simulink model "ES208A_CurrMeasArbn"  (R2013b)
settings: Solver=ode3  StartTime=0.0  StopTime=2  FixedStep=.000125  RelTol=1e-3
values from neighbouring files (symbols this model uses):
  CORRLNSTSCOMPCON1_ULS_U08 = DataDict.Constant    [ES208A_CurrMeasArbn_DataDict.m]
  CORRLNSTSCOMPCON2_ULS_U08 = DataDict.Constant    [ES208A_CurrMeasArbn_DataDict.m]
  CurrMeasArbnMaxStallCntr = DataDict.Calibration    [ES208A_CurrMeasArbn_DataDict.m]
  MOTCURRDAXQAXLIM_AMPR_F32 = DataDict.Constant    [ES208A_CurrMeasArbn_DataDict.m]
  ONEDIV3_ULS_F32 = DataDict.Constant    [ES208A_CurrMeasArbn_DataDict.m]
  ONEDIVSQRT3_ULS_F32 = DataDict.Constant    [ES208A_CurrMeasArbn_DataDict.m]
libraries: simulink x6
settings Model: Creator=hzy4g9  LastModifiedBy=hzy4g9
settings DebuggingCC: ParameterOverflowMsg=none

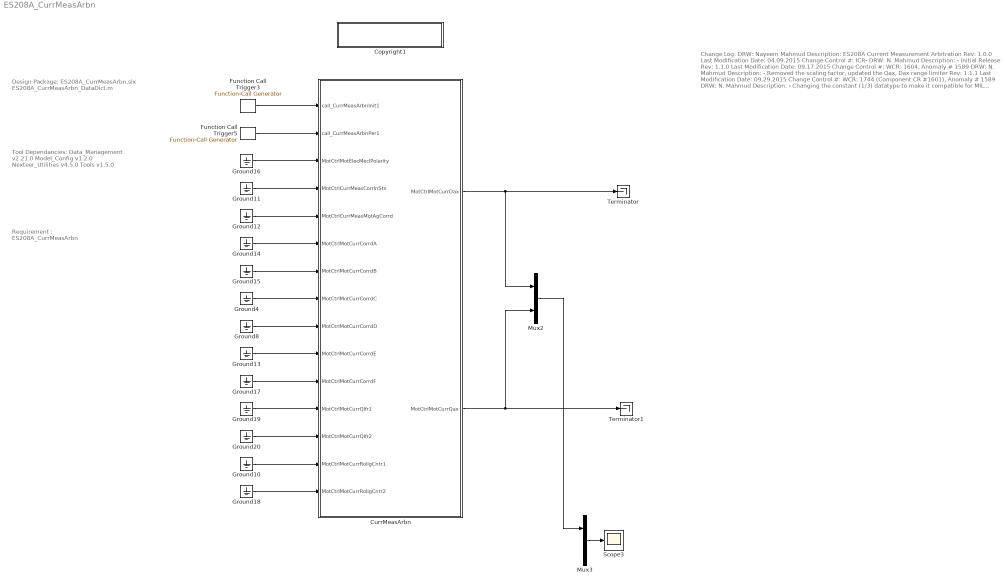
== system ES208A_CurrMeasArbn ==
  note: Design Package:
      |
      | ES208A_CurrMeasArbn.slx
      | ES208A_CurrMeasArbn_DataDict.m
  note: Tool Dependancies:
      |
      | Data_Management v2.21.0
      | Model_Config v1.2.0
      | Nexteer_Utilities v4.5.0
      | Tools v1.5.0
  note: Requirement :
      |
      | ES208A_CurrMeasArbn
  note: Change Log:
      |
      | DRW: Nayeem Mahmud
      | Description:
      | ES208A Current Measurement Arbitration
      |
      | Rev: 1.0.0
      | Last Modification Date: 04.09.2015
      | Change Control #: ICR-
      | DRW: N. Mahmud
      | Description:
      | - Initial Release
      |
      | Rev: 1.1.0
      | Last Modification Date: 09.17.2015
      | Change Control #: WCR: 1604, Anomaly # 1589
      | DRW: N. Mahmud
      | Description:
      | - Removed the scaling factor, updated the Qax, Dax range limiter
      |
      | Rev: 1.1.1
      | Last Modification Date: 09.29.2015
      | Change Control #: WCR: 1744 (Component CR #1601), Anomaly # 1589
      | DRW: N. Mahmud
      | Description:
      | - Changing the constant (1/3) datatype to make it compatible for MIL Testing.
      |
      |
      | Rev: 1.1.1
      | Last Modification Date: 09.29.2015
      | Change Control #: WCR: 1744 (Component CR #1601), Anomaly # 1589
      | DRW: N. Mahmud
      | Description:
      | - Changing the constant (1/3) datatype to make it compatible for MIL Testing.
      |
      |
      | Rev: 1.2.0
      | Last Modification Date: 10.16.2015
      | Change Control #: WCR: 2039 (Component CR #2011), Anomaly # 1965
      | DRW: N. Mahmud
      | Description:
      | - Requirement linkage between FR and the model has been corrected according the the MIL test review.
      | - Details can be found in Muragesh's email on 10.06.2015
      |
      |
      | Rev: 1.3.0
      | Last Modification Date: 03.15.2016
      | Change Control #: Anomaly # EA4#2989     Comp   EA4#4532	     WCR # EA4#4751
      | DRW: N. Mahmud
      | Description:
      | - Fixed the datatype mismatch on CurrMeasCorrlnSts connection
  Copyright1 : Subsystem  Description=|  mask(Copyright Information){none=on}
      | Copyright info block.                                               
      |                                                                     
      | Place copyright information at the top of every subsystem in design.
      mask prompts: none "No parameters"
      mask help: Place copyright information at the top of every subsystem in design.
      mask Display:
      | NxtrConf = 'Nexteer Confidential';
      | 
      | sys = bdroot; %handle for the current model ("system")
      | first = get_param(sys,'Created');
      | if(isempty(first))
      |     first = datestr(now,'yyyy');
      | else
      |     first = first(end-3:end);  %year is last four digits
      | end
      | 
      | last = get_param(sys,'LastModifiedDate');
      | if isempty(last)
      |     last = datestr(now,'yyyy');
      | else
      |     last = last(end-3:end);
      | end
      | 
      | if strcmp(first,last)
      |     fprintf('%s\nCopyright  %s Nexteer',NxtrConf,first);
      | else
      |     fprintf('%s\n%s%s-%s Nexteer',NxtrConf,char(169),first,last);
      | end
  CurrMeasArbn : Subsystem  RequirementInfo={} %GIDa_a1717183_1af4_4d60_b453_ff5ac2b3c2e1
  Function Call Trigger3 : simulink/Ports & Subsystems/Function-Call Generator  RequirementInfo={} %GIDa_b2c5acfa_4dcb_4ad4_8951_e2fcc0578f85  sample_time=0  numberOfIterations=1
  Function Call Trigger5 : simulink/Ports & Subsystems/Function-Call Generator  RequirementInfo={} %GIDa_0decdd2a_d3f7_4f78_a697_e4983ae5479f  sample_time=0.000125  numberOfIterations=1
  Ground{4,8,10..20} (13 alike) : Ground
  Mux2 : Mux  Inputs=2
  Mux3 : Mux  Inputs=2
  Scope3 : Scope
      settings: TimeRange=2  YMin=-70  YMax=70  SaveName=ScopeData6
  Terminator : Terminator
  Terminator1 : Terminator
  wires:
  Mux2/1 -> Mux3/1
  CurrMeasArbn/2(MotCtrlMotCurrQax) -> Mux2/2, Terminator1/1
  CurrMeasArbn/1(MotCtrlMotCurrDax) -> Terminator/1, Mux2/1
  Mux3/1 -> Scope3/1
  Function Call Trigger3/1 -> CurrMeasArbn/1(call_CurrMeasArbnInit1)
  Function Call Trigger5/1 -> CurrMeasArbn/2(call_CurrMeasArbnPer1)
  Ground18/1 -> CurrMeasArbn/15(MotCtrlMotCurrRollgCntr2)
  Ground20/1 -> CurrMeasArbn/13(MotCtrlMotCurrQlfr2)
  Ground10/1 -> CurrMeasArbn/14(MotCtrlMotCurrRollgCntr1)
  Ground14/1 -> CurrMeasArbn/6(MotCtrlMotCurrCorrdA)
  Ground19/1 -> CurrMeasArbn/12(MotCtrlMotCurrQlfr1)
  Ground11/1 -> CurrMeasArbn/4(MotCtrlCurrMeasCorrlnSts)
  Ground16/1 -> CurrMeasArbn/3(MotCtrlMotElecMeclPolarity)
  Ground12/1 -> CurrMeasArbn/5(MotCtrlCurrMeasMotAgCorrd)
  Ground4/1 -> CurrMeasArbn/8(MotCtrlMotCurrCorrdC)
  Ground17/1 -> CurrMeasArbn/11(MotCtrlMotCurrCorrdF)
  Ground8/1 -> CurrMeasArbn/9(MotCtrlMotCurrCorrdD)
  Ground13/1 -> CurrMeasArbn/10(MotCtrlMotCurrCorrdE)
  Ground15/1 -> CurrMeasArbn/7(MotCtrlMotCurrCorrdB)

== system ES208A_CurrMeasArbn/Copyright1 ==

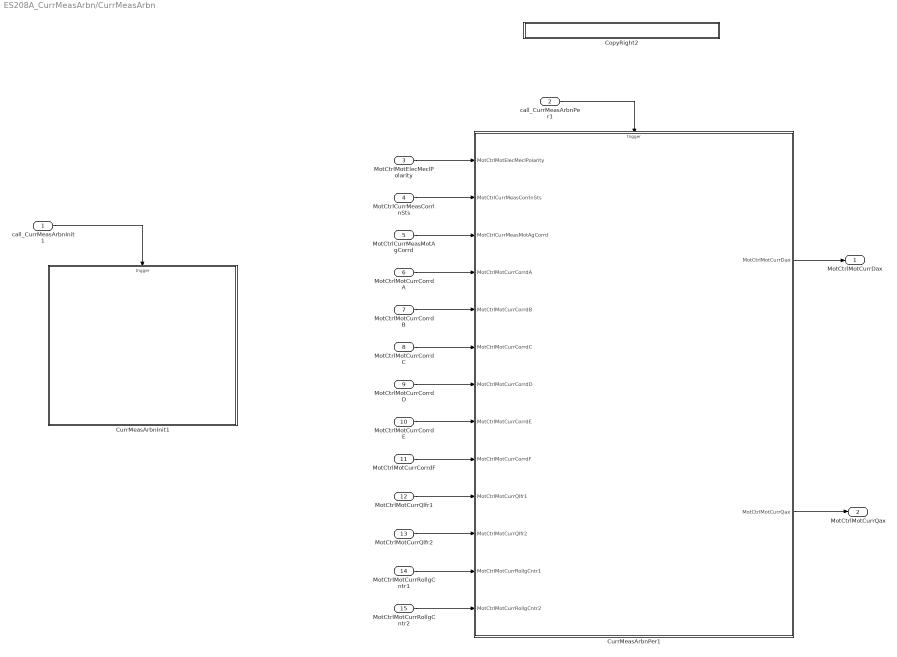
== system ES208A_CurrMeasArbn/CurrMeasArbn ==
  call_CurrMeasArbnInit1 : Inport
  call_CurrMeasArbnPer1 : Inport  Port=2
  MotCtrlMotElecMeclPolarity : Inport  RequirementInfo={'linktype_rmi_doors' '0000c363 (/ESG Group/FDD Module Requirements/EA4 Specific/ES208A CurrMeasArbn)' '#ES208A_200' 'true' 'REQ: ES208A_200' '' } %GIDa_2b3b6ccf_6739_4b84_95f8_6a6981087fde  Port=3
  MotCtrlCurrMeasCorrlnSts : Inport  RequirementInfo={'linktype_rmi_doors' '0000c363 (/ESG Group/FDD Module Requirements/EA4 Specific/ES208A CurrMeasArbn)' '#ES208A_205' 'true' 'REQ: ES208A_205' '' } %GIDa_b47cd3a1_346e_4c9b_a755_1899bf4f1f90  Port=4  OutDataTypeStr=uint16
  MotCtrlCurrMeasMotAgCorrd : Inport  RequirementInfo={'linktype_rmi_doors' '0000c363 (/ESG Group/FDD Module Requirements/EA4 Specific/ES208A CurrMeasArbn)' '#ES208A_202' 'true' 'REQ: ES208A_202' '' } %GIDa_3e28adf7_2d4b_4fb8_a0eb_8bdd2948163c  Port=5
  MotCtrlMotCurrCorrdA : Inport  RequirementInfo={'linktype_rmi_doors' '0000c363 (/ESG Group/FDD Module Requirements/EA4 Specific/ES208A CurrMeasArbn)' '#ES208A_104' 'true' 'REQ: ES208A_104' '' } %GIDa_fa60b5af_feb4_4057_8a17_b1f1cd5e1840  Port=6
  MotCtrlMotCurrCorrdB : Inport  RequirementInfo={'linktype_rmi_doors' '0000c363 (/ESG Group/FDD Module Requirements/EA4 Specific/ES208A CurrMeasArbn)' '#ES208A_103' 'true' 'REQ: ES208A_103' '' } %GIDa_236fb9c2_37b3_44dd_950c_8b8dc24ebe1f  Port=7
  MotCtrlMotCurrCorrdC : Inport  RequirementInfo={'linktype_rmi_doors' '0000c363 (/ESG Group/FDD Module Requirements/EA4 Specific/ES208A CurrMeasArbn)' '#ES208A_102' 'true' 'REQ: ES208A_102' '' } %GIDa_cb87798d_9ed2_4f24_a94d_155ef6f739fe  Port=8
  MotCtrlMotCurrCorrdD : Inport  RequirementInfo={'linktype_rmi_doors' '0000c363 (/ESG Group/FDD Module Requirements/EA4 Specific/ES208A CurrMeasArbn)' '#ES208A_101' 'true' 'REQ: ES208A_101' '' } %GIDa_061ae548_4f5f_4f77_9e99_bc9a7a97246f  Port=9
  MotCtrlMotCurrCorrdE : Inport  RequirementInfo={'linktype_rmi_doors' '0000c363 (/ESG Group/FDD Module Requirements/EA4 Specific/ES208A CurrMeasArbn)' '#ES208A_100' 'true' 'REQ: ES208A_100' '' } %GIDa_a1510a61_0232_4d8b_b15e_5251ba81e48f  Port=10
  MotCtrlMotCurrCorrdF : Inport  RequirementInfo={'linktype_rmi_doors' '0000c363 (/ESG Group/FDD Module Requirements/EA4 Specific/ES208A CurrMeasArbn)' '#ES208A_99' 'true' 'REQ: ES208A_99' '' } %GIDa_55e2ee94_269a_4388_9a08_e4c1affacd3d  Port=11
  MotCtrlMotCurrQlfr1 : Inport  RequirementInfo={'linktype_rmi_doors' '0000c363 (/ESG Group/FDD Module Requirements/EA4 Specific/ES208A CurrMeasArbn)' '#ES208A_215' 'true' 'REQ: ES208A_215' '' } %GIDa_d01b7b7a_10d2_4143_9f7b_655c2bbf76c3  Port=12
  MotCtrlMotCurrQlfr2 : Inport  RequirementInfo={'linktype_rmi_doors' '0000c363 (/ESG Group/FDD Module Requirements/EA4 Specific/ES208A CurrMeasArbn)' '#ES208A_214' 'true' 'REQ: ES208A_214' '' } %GIDa_a588847a_814e_4cd9_8192_8cc5b2289da5  Port=13
  MotCtrlMotCurrRollgCntr1 : Inport  RequirementInfo={'linktype_rmi_doors' '0000c363 (/ESG Group/FDD Module Requirements/EA4 Specific/ES208A CurrMeasArbn)' '#ES208A_213' 'true' 'REQ: ES208A_213' '' } %GIDa_81545b02_05c2_4ea8_b385_fe805407db0a  Port=14
  MotCtrlMotCurrRollgCntr2 : Inport  RequirementInfo={'linktype_rmi_doors' '0000c363 (/ESG Group/FDD Module Requirements/EA4 Specific/ES208A CurrMeasArbn)' '#ES208A_212' 'true' 'REQ: ES208A_212' '' } %GIDa_f58fb777_4bd7_43f0_8970_a93616277b47  Port=15
  CopyRight2 : Subsystem  Description=|  mask(Copyright Information){none=on}
      | Copyright info block.                                               
      |                                                                     
      | Place copyright information at the top of every subsystem in design.
      mask prompts: none "No parameters"
      mask help: Place copyright information at the top of every subsystem in design.
      mask Display:
      | NxtrConf = 'Nexteer Confidential';
      | 
      | sys = bdroot; %handle for the current model ("system")
      | first = get_param(sys,'Created');
      | first = first(end-3:end);  %year is last four digits
      | 
      | last = get_param(sys,'LastModifiedDate');
      | if isempty(last)
      |     last = datestr(now,'yyyy');
      | else
      |     last = last(end-3:end);
      | end
      | 
      | if strcmp(first,last)
      |     fprintf('%s -- Copyright %s Nexteer',NxtrConf,first)
      | else
      |     fprintf('%s -- %s%s- %s Nexteer',NxtrConf,char(169),first,last)
      | end
  CurrMeasArbnInit1 : Subsystem  RequirementInfo={'linktype_rmi_doors' '0000c363 (/ESG Group/FDD Module Requirements/EA4 Specific/ES208A CurrMeasArbn)' '#ES208A_216' 'true' 'REQ: ES208A_216' '' } %GIDa_4d08f95b_63fa_42b7_bb43_10901df62bca
  CurrMeasArbnPer1 : Subsystem  RequirementInfo={'linktype_rmi_doors' '0000c363 (/ESG Group/FDD Module Requirements/EA4 Specific/ES208A CurrMeasArbn)' '#ES208A_216' 'true' 'REQ: ES208A_216' '' } %GIDa_5d0a6b13_94ef_43df_a64b_8db993e8cc82
  MotCtrlMotCurrDax : Outport  RequirementInfo={'linktype_rmi_doors' '0000c363 (/ESG Group/FDD Module Requirements/EA4 Specific/ES208A CurrMeasArbn)' '#ES208A_204' 'true' 'REQ: ES208A_204' '' } %GIDa_641f96e7_6a3f_402c_952a_c727130605fe
  MotCtrlMotCurrQax : Outport  RequirementInfo={'linktype_rmi_doors' '0000c363 (/ESG Group/FDD Module Requirements/EA4 Specific/ES208A CurrMeasArbn)' '#ES208A_206' 'true' 'REQ: ES208A_206' '' } %GIDa_55e00c49_dae8_43a4_8cfe_81b053089442  Port=2
  wires:
  CurrMeasArbnPer1/1(MotCtrlMotCurrDax) -> MotCtrlMotCurrDax/1
  CurrMeasArbnPer1/2(MotCtrlMotCurrQax) -> MotCtrlMotCurrQax/1
  call_CurrMeasArbnPer1/1 -> CurrMeasArbnPer1/Trigger
  MotCtrlMotElecMeclPolarity/1 -> CurrMeasArbnPer1/1(MotCtrlMotElecMeclPolarity)
  MotCtrlCurrMeasCorrlnSts/1 -> CurrMeasArbnPer1/2(MotCtrlCurrMeasCorrlnSts)
  MotCtrlCurrMeasMotAgCorrd/1 -> CurrMeasArbnPer1/3(MotCtrlCurrMeasMotAgCorrd)
  MotCtrlMotCurrCorrdA/1 -> CurrMeasArbnPer1/4(MotCtrlMotCurrCorrdA)
  MotCtrlMotCurrCorrdB/1 -> CurrMeasArbnPer1/5(MotCtrlMotCurrCorrdB)
  MotCtrlMotCurrCorrdC/1 -> CurrMeasArbnPer1/6(MotCtrlMotCurrCorrdC)
  MotCtrlMotCurrCorrdD/1 -> CurrMeasArbnPer1/7(MotCtrlMotCurrCorrdD)
  MotCtrlMotCurrCorrdE/1 -> CurrMeasArbnPer1/8(MotCtrlMotCurrCorrdE)
  MotCtrlMotCurrCorrdF/1 -> CurrMeasArbnPer1/9(MotCtrlMotCurrCorrdF)
  MotCtrlMotCurrQlfr1/1 -> CurrMeasArbnPer1/10(MotCtrlMotCurrQlfr1)
  MotCtrlMotCurrQlfr2/1 -> CurrMeasArbnPer1/11(MotCtrlMotCurrQlfr2)
  MotCtrlMotCurrRollgCntr1/1 -> CurrMeasArbnPer1/12(MotCtrlMotCurrRollgCntr1)
  MotCtrlMotCurrRollgCntr2/1 -> CurrMeasArbnPer1/13(MotCtrlMotCurrRollgCntr2)
  call_CurrMeasArbnInit1/1 -> CurrMeasArbnInit1/Trigger

== system ES208A_CurrMeasArbn/CurrMeasArbn/CopyRight2 ==

== system ES208A_CurrMeasArbn/CurrMeasArbn/CurrMeasArbnInit1 ==
  note: Init function is added to have a RTE function associated with the periodic
      | which runs at motor control ISR rate so that Calibrations and PIMs can be
      | initialized/configured through RTE
  Trigger : TriggerPort  TriggerType=function-call  PortDimensions=1

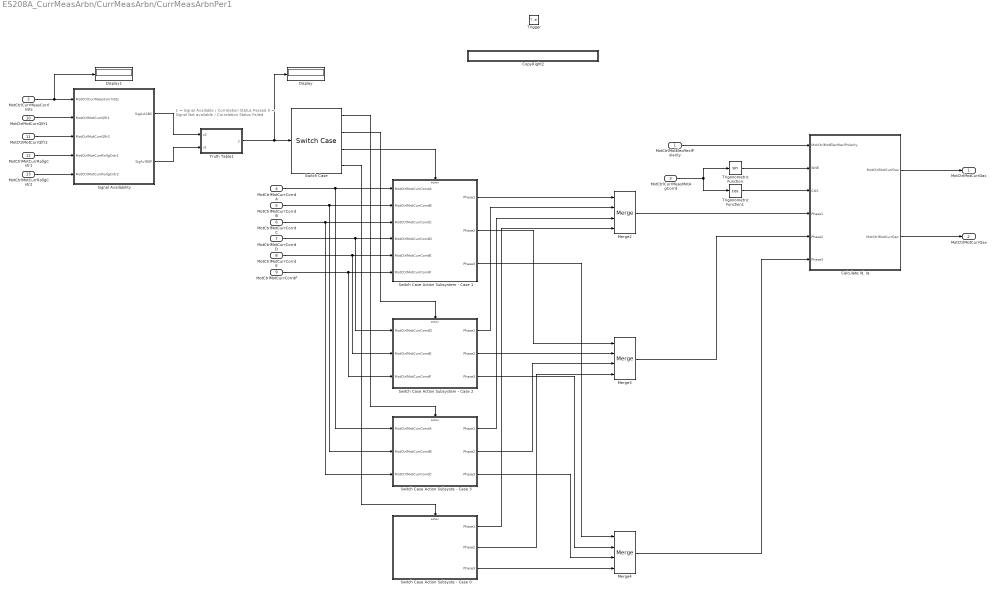
== system ES208A_CurrMeasArbn/CurrMeasArbn/CurrMeasArbnPer1 ==
  note: 1 = Signal Available / Correlation Status Passed
      | 0 = Signal Not available / Correlation Status Failed
  MotCtrlMotElecMeclPolarity : Inport  RequirementInfo={} %GIDa_236c7770_dbe0_4d6b_854a_af419427730c
  MotCtrlCurrMeasCorrlnSts : Inport  RequirementInfo={} %GIDa_5f0ff581_beb2_45c0_96fc_3ae60b8cafd0  Port=2
  MotCtrlCurrMeasMotAgCorrd : Inport  Port=3  OutDataTypeStr=single
  MotCtrlMotCurrCorrdA : Inport  RequirementInfo={} %GIDa_f9a6d725_8597_45da_8d5a_d49e87f1c418  Port=4
  MotCtrlMotCurrCorrdB : Inport  RequirementInfo={} %GIDa_4ecfd322_1f8c_4f95_b72b_4a4f2c3592db  Port=5
  MotCtrlMotCurrCorrdC : Inport  RequirementInfo={} %GIDa_50682985_192f_42e9_ab67_18d9d790db6a  Port=6
  MotCtrlMotCurrCorrdD : Inport  RequirementInfo={} %GIDa_08227d3c_7fbb_46ed_9d72_22bcb1c5ff3a  Port=7
  MotCtrlMotCurrCorrdE : Inport  RequirementInfo={} %GIDa_5724e0f4_ed90_4089_ab16_14491ea93933  Port=8
  MotCtrlMotCurrCorrdF : Inport  RequirementInfo={} %GIDa_7a043740_7caa_40bd_b933_0baae6bc5fb0  Port=9
  MotCtrlMotCurrQlfr1 : Inport  RequirementInfo={} %GIDa_d0b4e530_bfd9_4c60_aa9a_209d86ff3bd1  Port=10
  MotCtrlMotCurrQlfr2 : Inport  RequirementInfo={} %GIDa_775a9752_c098_48a0_adc4_e5952c0b608a  Port=11
  MotCtrlMotCurrRollgCntr1 : Inport  RequirementInfo={} %GIDa_059ee444_07c8_42c9_bb13_b03c4afc962a  Port=12
  MotCtrlMotCurrRollgCntr2 : Inport  RequirementInfo={} %GIDa_23ffabf9_7016_4a97_b10a_a8e5452610f9  Port=13  OutDataTypeStr=uint8
  Trigger : TriggerPort  TriggerType=function-call  PortDimensions=1
  "Calculate Id, Iq" : Subsystem  RequirementInfo={'linktype_rmi_doors' '0000c363 (/ESG Group/FDD Module Requirements/EA4 Specific/ES208A CurrMeasArbn)' '#ES208A_15' 'true' 'REQ: ES208A_15' '' ; 'linktype_rmi_doors' '0000c363 (/ESG Group/FDD Module Requirements/EA4 Specific/ES208A CurrMeasArbn)' '#ES208A_221' 'true' 'REQ: ES208A_221' '' } %GIDa_d3675425_55ad_4442_a97f_0532e8744e77
  CopyRight2 : Subsystem  Description=|  mask(Copyright Information){none=on}
      | Copyright info block.                                               
      |                                                                     
      | Place copyright information at the top of every subsystem in design.
      mask prompts: none "No parameters"
      mask help: Place copyright information at the top of every subsystem in design.
      mask Display:
      | NxtrConf = 'Nexteer Confidential';
      | 
      | sys = bdroot; %handle for the current model ("system")
      | first = get_param(sys,'Created');
      | first = first(end-3:end);  %year is last four digits
      | 
      | last = get_param(sys,'LastModifiedDate');
      | if isempty(last)
      |     last = datestr(now,'yyyy');
      | else
      |     last = last(end-3:end);
      | end
      | 
      | if strcmp(first,last)
      |     fprintf('%s -- Copyright %s Nexteer',NxtrConf,first)
      | else
      |     fprintf('%s -- %s%s- %s Nexteer',NxtrConf,char(169),first,last)
      | end
  Display : Display
  Display1 : Display
  Merge2 : Merge  Inputs=4
  Merge3 : Merge  Inputs=4
  Merge4 : Merge  Inputs=4
  Signal Availability : Subsystem  RequirementInfo={} %GIDa_5e4be01c_85da_4430_af9b_2a4846b816f0
  Switch Case : SwitchCase  CaseConditions={3,2,1}
  Switch Case Action Subsyste - Case 0 : Subsystem  RequirementInfo={'linktype_rmi_doors' '0000c363 (/ESG Group/FDD Module Requirements/EA4 Specific/ES208A CurrMeasArbn)' '#ES208A_220' 'true' 'REQ: ES208A_220' '' } %GIDa_4f294f1a_407e_4985_88ae_1f48918d334e  TreatAsAtomicUnit=on
  Switch Case Action Subsyste - Case 3 : Subsystem  RequirementInfo={'linktype_rmi_doors' '0000c363 (/ESG Group/FDD Module Requirements/EA4 Specific/ES208A CurrMeasArbn)' '#ES208A_217' 'true' 'REQ: ES208A_217' '' } %GIDa_710d68b6_e234_43e9_bbdb_b14f4ce7fdcf  TreatAsAtomicUnit=on
  Switch Case Action Subsystem - Case 1 : Subsystem  RequirementInfo={'linktype_rmi_doors' '0000c363 (/ESG Group/FDD Module Requirements/EA4 Specific/ES208A CurrMeasArbn)' '#ES208A_211' 'true' 'REQ: ES208A_211' '' } %GIDa_4f02c82c_3123_42cc_bef6_8026bf4aaa33  TreatAsAtomicUnit=on
  Switch Case Action Subsystem - Case 2 : Subsystem  RequirementInfo={'linktype_rmi_doors' '0000c363 (/ESG Group/FDD Module Requirements/EA4 Specific/ES208A CurrMeasArbn)' '#ES208A_218' 'true' 'REQ: ES208A_218' '' } %GIDa_61ae6b1b_e240_4075_bddf_edb8f2fb6854  TreatAsAtomicUnit=on
  Trigonometric Function : Trigonometry
  Trigonometric Function1 : Trigonometry  Operator=cos
  Truth Table1 : Truth Table  TreatAsAtomicUnit=on
  MotCtrlMotCurrDax : Outport  RequirementInfo={} %GIDa_fc90444e_e698_458a_bc45_6a75ea4d8c72
  MotCtrlMotCurrQax : Outport  RequirementInfo={} %GIDa_65000aaa_3595_4279_a6c5_6d4c8a6042b5  Port=2
  wires:
  Truth Table1/1(y) -> Display/1, Switch Case/1
  MotCtrlCurrMeasMotAgCorrd/1 -> Trigonometric Function1/1, Trigonometric Function/1
  Switch Case/3 -> Switch Case Action Subsystem - Case 1/Action
  Switch Case/2 -> Switch Case Action Subsystem - Case 2/Action
  MotCtrlCurrMeasCorrlnSts/1 -> Signal Availability/1(MotCtrlCurrMeasCorrlnSts), Display1/1
  MotCtrlMotCurrQlfr2/1 -> Signal Availability/3(MotCtrlMotCurrQlfr2)
  MotCtrlMotCurrRollgCntr2/1 -> Signal Availability/5(MotCtrlMotCurrRollgCntr2)
  MotCtrlMotCurrQlfr1/1 -> Signal Availability/2(MotCtrlMotCurrQlfr1)
  MotCtrlMotCurrRollgCntr1/1 -> Signal Availability/4(MotCtrlMotCurrRollgCntr1)
  Signal Availability/1(SigAvlABC) -> Truth Table1/1(u2)
  Signal Availability/2("SigAvlDEF ") -> Truth Table1/2(u1)
  Switch Case/4 -> Switch Case Action Subsyste - Case 0/Action
  Switch Case/1 -> Switch Case Action Subsyste - Case 3/Action
  MotCtrlMotCurrCorrdC/1 -> Switch Case Action Subsyste - Case 3/3(MotCtrlMotCurrCorrdC), Switch Case Action Subsystem - Case 1/3(MotCtrlMotCurrCorrdC)
  MotCtrlMotCurrCorrdB/1 -> Switch Case Action Subsyste - Case 3/2(MotCtrlMotCurrCorrdB), Switch Case Action Subsystem - Case 1/2(MotCtrlMotCurrCorrdB)
  MotCtrlMotCurrCorrdA/1 -> Switch Case Action Subsyste - Case 3/1(MotCtrlMotCurrCorrdA), Switch Case Action Subsystem - Case 1/1(MotCtrlMotCurrCorrdA)
  MotCtrlMotCurrCorrdF/1 -> Switch Case Action Subsystem - Case 2/3(MotCtrlMotCurrCorrdF), Switch Case Action Subsystem - Case 1/6(MotCtrlMotCurrCorrdF)
  MotCtrlMotCurrCorrdD/1 -> Switch Case Action Subsystem - Case 2/1(MotCtrlMotCurrCorrdD), Switch Case Action Subsystem - Case 1/4(MotCtrlMotCurrCorrdD)
  MotCtrlMotCurrCorrdE/1 -> Switch Case Action Subsystem - Case 2/2(MotCtrlMotCurrCorrdE), Switch Case Action Subsystem - Case 1/5(MotCtrlMotCurrCorrdE)
  Switch Case Action Subsystem - Case 1/1(Phase1) -> Merge2/1
  Switch Case Action Subsystem - Case 2/1(Phase1) -> Merge2/2
  Switch Case Action Subsyste - Case 3/1(Phase1) -> Merge2/3
  Switch Case Action Subsyste - Case 0/1(Phase1) -> Merge2/4
  Switch Case Action Subsystem - Case 1/2(Phase2) -> Merge3/1
  Switch Case Action Subsystem - Case 2/2(Phase2) -> Merge3/2
  Switch Case Action Subsyste - Case 3/2(Phase2) -> Merge3/3
  Switch Case Action Subsyste - Case 0/2(Phase2) -> Merge3/4
  Switch Case Action Subsystem - Case 1/3(Phase3) -> Merge4/1
  Switch Case Action Subsystem - Case 2/3(Phase3) -> Merge4/2
  Switch Case Action Subsyste - Case 3/3(Phase3) -> Merge4/3
  Switch Case Action Subsyste - Case 0/3(Phase3) -> Merge4/4
  "Calculate Id, Iq"/1(MotCtrlMotCurrDax) -> MotCtrlMotCurrDax/1
  "Calculate Id, Iq"/2(MotCtrlMotCurrQax) -> MotCtrlMotCurrQax/1
  Trigonometric Function/1 -> "Calculate Id, Iq"/2(SINE)
  Trigonometric Function1/1 -> "Calculate Id, Iq"/3(COS)
  MotCtrlMotElecMeclPolarity/1 -> "Calculate Id, Iq"/1(MotCtrlMotElecMeclPolarity)
  Merge2/1 -> "Calculate Id, Iq"/4(Phase1)
  Merge3/1 -> "Calculate Id, Iq"/5(Phase2)
  Merge4/1 -> "Calculate Id, Iq"/6(Phase3)

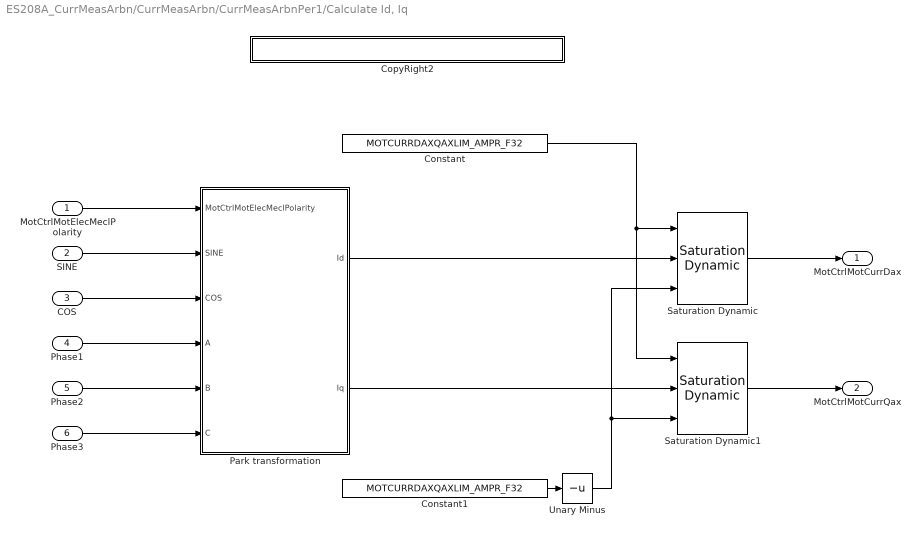
== system ES208A_CurrMeasArbn/CurrMeasArbn/CurrMeasArbnPer1/Calculate Id, Iq ==
  MotCtrlMotElecMeclPolarity : Inport  RequirementInfo={} %GIDa_f0c87258_af0d_44ef_b166_709dccf31a80
  SINE : Inport  Port=2
  COS : Inport  Port=3
  Phase1 : Inport  Port=4  OutDataTypeStr=single
  Phase2 : Inport  Port=5  OutDataTypeStr=single
  Phase3 : Inport  Port=6  OutDataTypeStr=single
  Constant : Constant  Value=MOTCURRDAXQAXLIM_AMPR_F32
  Constant1 : Constant  Value=MOTCURRDAXQAXLIM_AMPR_F32
  CopyRight2 : Subsystem  Description=|  mask(Copyright Information){none=on}
      | Copyright info block.                                               
      |                                                                     
      | Place copyright information at the top of every subsystem in design.
      mask prompts: none "No parameters"
      mask help: Place copyright information at the top of every subsystem in design.
      mask Display:
      | NxtrConf = 'Nexteer Confidential';
      | 
      | sys = bdroot; %handle for the current model ("system")
      | first = get_param(sys,'Created');
      | first = first(end-3:end);  %year is last four digits
      | 
      | last = get_param(sys,'LastModifiedDate');
      | if isempty(last)
      |     last = datestr(now,'yyyy');
      | else
      |     last = last(end-3:end);
      | end
      | 
      | if strcmp(first,last)
      |     fprintf('%s -- Copyright %s Nexteer',NxtrConf,first)
      | else
      |     fprintf('%s -- %s%s- %s Nexteer',NxtrConf,char(169),first,last)
      | end
  Park transformation : Subsystem  RequirementInfo={'linktype_rmi_doors' '0000c363 (/ESG Group/FDD Module Requirements/EA4 Specific/ES208A CurrMeasArbn)' '#ES208A_221' 'true' 'REQ: ES208A_221' '' } %GIDa_d3ede396_e304_4918_89ce_5b6c0de97769
  Saturation Dynamic : simulink/Discontinuities/Saturation Dynamic  RequirementInfo={'linktype_rmi_doors' '0000c363 (/ESG Group/FDD Module Requirements/EA4 Specific/ES208A CurrMeasArbn)' '#ES208A_222' 'true' 'REQ: ES208A_222' '' } %GIDa_6e2e1fe4_dfc6_46e0_b1ff_e247798a13b4  OutMin=[]  OutMax=[]  OutDataTypeStr=Inherit: Same as second input  OutDataType=fixdt(1, 16)  OutScaling=2^-10  DoSatur=off
  Saturation Dynamic1 : simulink/Discontinuities/Saturation Dynamic  RequirementInfo={'linktype_rmi_doors' '0000c363 (/ESG Group/FDD Module Requirements/EA4 Specific/ES208A CurrMeasArbn)' '#ES208A_222' 'true' 'REQ: ES208A_222' '' } %GIDa_ef7f06fc_ceb7_4b34_a03b_affe5dfaca83  OutMin=[]  OutMax=[]  OutDataTypeStr=Inherit: Same as second input  OutDataType=fixdt(1, 16)  OutScaling=2^-10  DoSatur=off
  Unary Minus : UnaryMinus
  MotCtrlMotCurrDax : Outport
  MotCtrlMotCurrQax : Outport  Port=2
  wires:
  Phase2/1 -> Park transformation/5(B)
  Phase3/1 -> Park transformation/6(C)
  Phase1/1 -> Park transformation/4(A)
  MotCtrlMotElecMeclPolarity/1 -> Park transformation/1(MotCtrlMotElecMeclPolarity)
  SINE/1 -> Park transformation/2(SINE)
  COS/1 -> Park transformation/3(COS)
  Park transformation/1(Id) -> Saturation Dynamic/2
  Park transformation/2(Iq) -> Saturation Dynamic1/2
  Saturation Dynamic/1 -> MotCtrlMotCurrDax/1
  Saturation Dynamic1/1 -> MotCtrlMotCurrQax/1
  Constant/1 -> Saturation Dynamic/1, Saturation Dynamic1/1
  Unary Minus/1 -> Saturation Dynamic/3, Saturation Dynamic1/3
  Constant1/1 -> Unary Minus/1

== system ES208A_CurrMeasArbn/CurrMeasArbn/CurrMeasArbnPer1/CopyRight2 ==

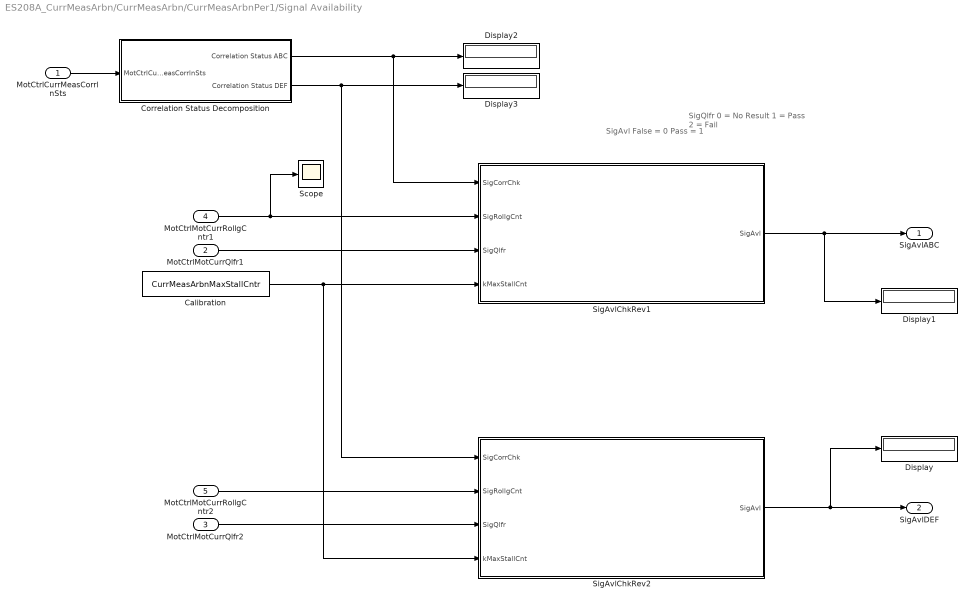
== system ES208A_CurrMeasArbn/CurrMeasArbn/CurrMeasArbnPer1/Signal Availability ==
  note: SigQlfr
      | 0 = No Result
      | 1 = Pass
      | 2 = Fail
  note: SigAvl
      | False = 0
      | Pass = 1
  MotCtrlCurrMeasCorrlnSts : Inport
  MotCtrlMotCurrQlfr1 : Inport  RequirementInfo={} %GIDa_edd0a4a8_ec9a_4294_bd7b_dc00380f4e82  Port=2
  MotCtrlMotCurrQlfr2 : Inport  RequirementInfo={} %GIDa_39258a34_15c4_42b2_b2a5_87a9df44d1d3  Port=3
  MotCtrlMotCurrRollgCntr1 : Inport  RequirementInfo={} %GIDa_9fc2b2d5_9d4a_4481_bff5_db7bbf1f5598  Port=4
  MotCtrlMotCurrRollgCntr2 : Inport  RequirementInfo={} %GIDa_1cde4ce6_8634_4cd8_b985_cde8bd6e892e  Port=5
  Calibration : Constant  Value=CurrMeasArbnMaxStallCntr
  "Correlation Status Decomposition " : Subsystem  RequirementInfo={'linktype_rmi_doors' '0000c363 (/ESG Group/FDD Module Requirements/EA4 Specific/ES208A CurrMeasArbn)' '#ES208A_135' 'true' 'REQ: ES208A_135' '' ; 'linktype_rmi_doors' '0000c363 (/ESG Group/FDD Module Requirements/EA4 Specific/ES208A CurrMeasArbn)' '#ES208A_219' 'true' 'REQ: ES208A_219' '' } %GIDa_c140fad4_ae0f_42b6_91b3_b7b2268b2aab
  Display{,1..3} (4 alike) : Display
  Scope : Scope
  SigAvlChkRev1 : Subsystem  RequirementInfo={'linktype_rmi_doors' '0000c363 (/ESG Group/FDD Module Requirements/EA4 Specific/ES208A CurrMeasArbn)' '#ES208A_135' 'true' 'REQ: ES208A_135' '' } %GIDa_b2a9f5a1_8dd0_41b9_a883_77a286bcb317  TreatAsAtomicUnit=on
  SigAvlChkRev2 : Subsystem  RequirementInfo={'linktype_rmi_doors' '0000c363 (/ESG Group/FDD Module Requirements/EA4 Specific/ES208A CurrMeasArbn)' '#ES208A_219' 'true' 'REQ: ES208A_219' '' } %GIDa_bf4ef0a2_bb1f_46f7_985b_0b0c9d147fc2  TreatAsAtomicUnit=on
  SigAvlABC : Outport
  "SigAvlDEF " : Outport  Port=2
  wires:
  MotCtrlCurrMeasCorrlnSts/1 -> "Correlation Status Decomposition "/1(MotCtrlCurrMeasCorrlnSts)
  "Correlation Status Decomposition "/1(Correlation Status ABC) -> SigAvlChkRev1/1(SigCorrChk), Display2/1
  MotCtrlMotCurrRollgCntr1/1 -> SigAvlChkRev1/2(SigRollgCnt), Scope/1
  MotCtrlMotCurrQlfr1/1 -> SigAvlChkRev1/3(SigQlfr)
  "Correlation Status Decomposition "/2(Correlation Status DEF) -> SigAvlChkRev2/1(SigCorrChk), Display3/1
  MotCtrlMotCurrRollgCntr2/1 -> SigAvlChkRev2/2(SigRollgCnt)
  MotCtrlMotCurrQlfr2/1 -> SigAvlChkRev2/3(SigQlfr)
  Calibration/1 -> SigAvlChkRev2/4(kMaxStallCnt), SigAvlChkRev1/4(kMaxStallCnt)
  SigAvlChkRev2/1(SigAvl) -> Display/1, "SigAvlDEF "/1
  SigAvlChkRev1/1(SigAvl) -> SigAvlABC/1, Display1/1

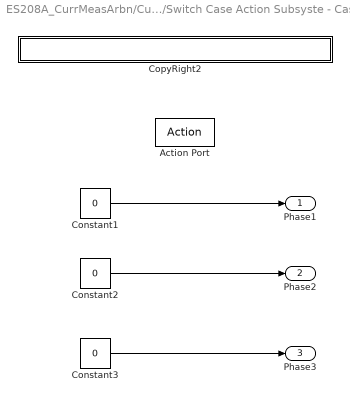
== system ES208A_CurrMeasArbn/CurrMeasArbn/CurrMeasArbnPer1/Switch Case Action Subsyste - Case 0 ==
  Action Port : ActionPort  ActionType=default
  Constant1 : Constant  Value=0  OutDataTypeStr=single
  Constant2 : Constant  Value=0  OutDataTypeStr=single
  Constant3 : Constant  Value=0  OutDataTypeStr=single
  CopyRight2 : Subsystem  Description=|  mask(Copyright Information){none=on}
      | Copyright info block.                                               
      |                                                                     
      | Place copyright information at the top of every subsystem in design.
      mask prompts: none "No parameters"
      mask help: Place copyright information at the top of every subsystem in design.
      mask Display:
      | NxtrConf = 'Nexteer Confidential';
      | 
      | sys = bdroot; %handle for the current model ("system")
      | first = get_param(sys,'Created');
      | first = first(end-3:end);  %year is last four digits
      | 
      | last = get_param(sys,'LastModifiedDate');
      | if isempty(last)
      |     last = datestr(now,'yyyy');
      | else
      |     last = last(end-3:end);
      | end
      | 
      | if strcmp(first,last)
      |     fprintf('%s -- Copyright %s Nexteer',NxtrConf,first)
      | else
      |     fprintf('%s -- %s%s- %s Nexteer',NxtrConf,char(169),first,last)
      | end
  Phase1 : Outport
  Phase2 : Outport  Port=2
  Phase3 : Outport  Port=3
  wires:
  Constant2/1 -> Phase2/1
  Constant1/1 -> Phase1/1
  Constant3/1 -> Phase3/1

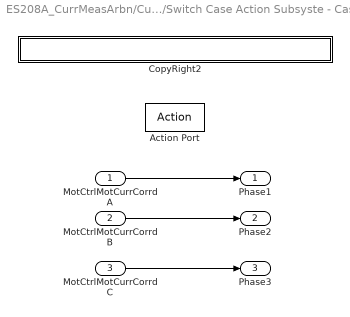
== system ES208A_CurrMeasArbn/CurrMeasArbn/CurrMeasArbnPer1/Switch Case Action Subsyste - Case 3 ==
  MotCtrlMotCurrCorrdA : Inport
  MotCtrlMotCurrCorrdB : Inport  Port=2
  MotCtrlMotCurrCorrdC : Inport  Port=3
  Action Port : ActionPort  ActionType=case
  CopyRight2 : Subsystem  Description=|  mask(Copyright Information){none=on}
      | Copyright info block.                                               
      |                                                                     
      | Place copyright information at the top of every subsystem in design.
      mask prompts: none "No parameters"
      mask help: Place copyright information at the top of every subsystem in design.
      mask Display:
      | NxtrConf = 'Nexteer Confidential';
      | 
      | sys = bdroot; %handle for the current model ("system")
      | first = get_param(sys,'Created');
      | first = first(end-3:end);  %year is last four digits
      | 
      | last = get_param(sys,'LastModifiedDate');
      | if isempty(last)
      |     last = datestr(now,'yyyy');
      | else
      |     last = last(end-3:end);
      | end
      | 
      | if strcmp(first,last)
      |     fprintf('%s -- Copyright %s Nexteer',NxtrConf,first)
      | else
      |     fprintf('%s -- %s%s- %s Nexteer',NxtrConf,char(169),first,last)
      | end
  Phase1 : Outport
  Phase2 : Outport  Port=2
  Phase3 : Outport  Port=3
  wires:
  MotCtrlMotCurrCorrdC/1 -> Phase3/1
  MotCtrlMotCurrCorrdB/1 -> Phase2/1
  MotCtrlMotCurrCorrdA/1 -> Phase1/1

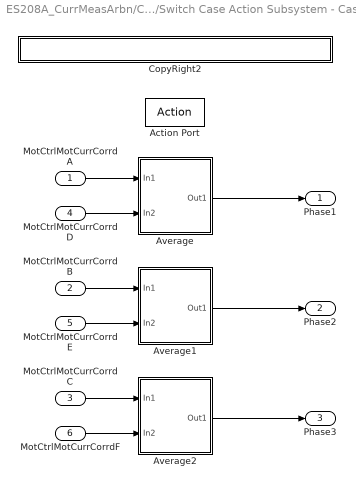
== system ES208A_CurrMeasArbn/CurrMeasArbn/CurrMeasArbnPer1/Switch Case Action Subsystem - Case 1 ==
  MotCtrlMotCurrCorrdA : Inport
  MotCtrlMotCurrCorrdB : Inport  Port=2
  MotCtrlMotCurrCorrdC : Inport  Port=3
  MotCtrlMotCurrCorrdD : Inport  Port=4
  MotCtrlMotCurrCorrdE : Inport  Port=5
  MotCtrlMotCurrCorrdF : Inport  Port=6
  Action Port : ActionPort  ActionType=case
  Average : Subsystem
  Average1 : Subsystem
  Average2 : Subsystem
  CopyRight2 : Subsystem  Description=|  mask(Copyright Information){none=on}
      | Copyright info block.                                               
      |                                                                     
      | Place copyright information at the top of every subsystem in design.
      mask prompts: none "No parameters"
      mask help: Place copyright information at the top of every subsystem in design.
      mask Display:
      | NxtrConf = 'Nexteer Confidential';
      | 
      | sys = bdroot; %handle for the current model ("system")
      | first = get_param(sys,'Created');
      | first = first(end-3:end);  %year is last four digits
      | 
      | last = get_param(sys,'LastModifiedDate');
      | if isempty(last)
      |     last = datestr(now,'yyyy');
      | else
      |     last = last(end-3:end);
      | end
      | 
      | if strcmp(first,last)
      |     fprintf('%s -- Copyright %s Nexteer',NxtrConf,first)
      | else
      |     fprintf('%s -- %s%s- %s Nexteer',NxtrConf,char(169),first,last)
      | end
  Phase1 : Outport
  Phase2 : Outport  Port=2
  Phase3 : Outport  Port=3
  wires:
  MotCtrlMotCurrCorrdA/1 -> Average/1(In1)
  MotCtrlMotCurrCorrdD/1 -> Average/2(In2)
  MotCtrlMotCurrCorrdE/1 -> Average1/2(In2)
  MotCtrlMotCurrCorrdB/1 -> Average1/1(In1)
  MotCtrlMotCurrCorrdF/1 -> Average2/2(In2)
  MotCtrlMotCurrCorrdC/1 -> Average2/1(In1)
  Average/1(Out1) -> Phase1/1
  Average2/1(Out1) -> Phase3/1
  Average1/1(Out1) -> Phase2/1

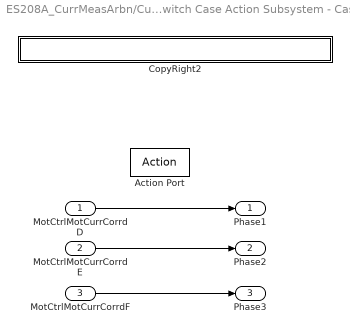
== system ES208A_CurrMeasArbn/CurrMeasArbn/CurrMeasArbnPer1/Switch Case Action Subsystem - Case 2 ==
  MotCtrlMotCurrCorrdD : Inport
  MotCtrlMotCurrCorrdE : Inport  Port=2
  MotCtrlMotCurrCorrdF : Inport  Port=3
  Action Port : ActionPort  ActionType=case
  CopyRight2 : Subsystem  Description=|  mask(Copyright Information){none=on}
      | Copyright info block.                                               
      |                                                                     
      | Place copyright information at the top of every subsystem in design.
      mask prompts: none "No parameters"
      mask help: Place copyright information at the top of every subsystem in design.
      mask Display:
      | NxtrConf = 'Nexteer Confidential';
      | 
      | sys = bdroot; %handle for the current model ("system")
      | first = get_param(sys,'Created');
      | first = first(end-3:end);  %year is last four digits
      | 
      | last = get_param(sys,'LastModifiedDate');
      | if isempty(last)
      |     last = datestr(now,'yyyy');
      | else
      |     last = last(end-3:end);
      | end
      | 
      | if strcmp(first,last)
      |     fprintf('%s -- Copyright %s Nexteer',NxtrConf,first)
      | else
      |     fprintf('%s -- %s%s- %s Nexteer',NxtrConf,char(169),first,last)
      | end
  Phase1 : Outport
  Phase2 : Outport  Port=2
  Phase3 : Outport  Port=3
  wires:
  MotCtrlMotCurrCorrdF/1 -> Phase3/1
  MotCtrlMotCurrCorrdE/1 -> Phase2/1
  MotCtrlMotCurrCorrdD/1 -> Phase1/1

== system ES208A_CurrMeasArbn/CurrMeasArbn/CurrMeasArbnPer1/Calculate Id, Iq/CopyRight2 ==

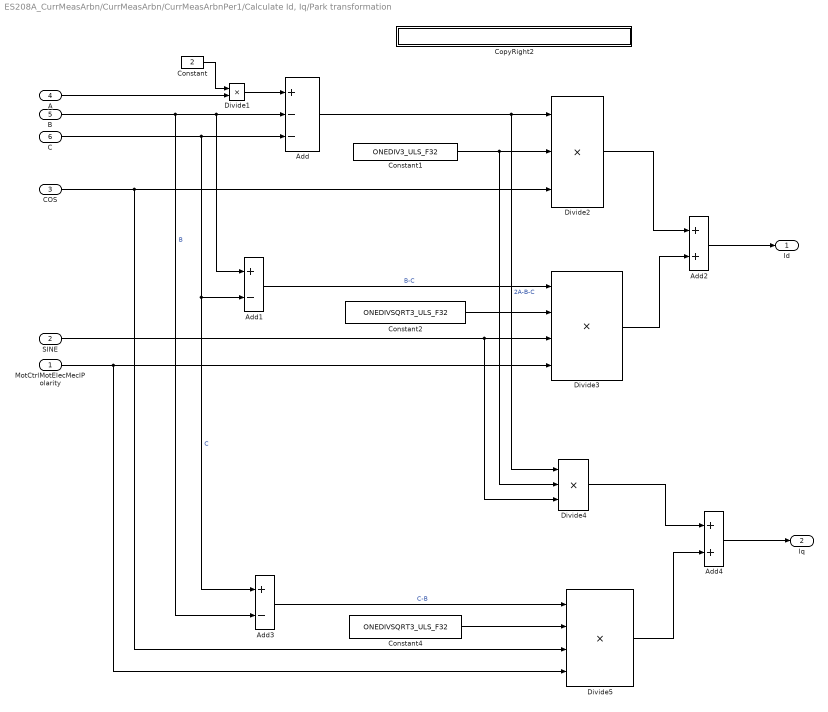
== system ES208A_CurrMeasArbn/CurrMeasArbn/CurrMeasArbnPer1/Calculate Id, Iq/Park transformation ==
  MotCtrlMotElecMeclPolarity : Inport  RequirementInfo={} %GIDa_caabb2a1_c069_4e98_81e6_8ee78cb88430
  SINE : Inport  Port=2
  COS : Inport  Port=3
  A : Inport  Port=4
  B : Inport  Port=5
  C : Inport  Port=6
  Add : Sum  Inputs=+--
  Add1 : Sum  Inputs=+-
  Add2 : Sum
  Add3 : Sum  Inputs=+-
  Add4 : Sum
  Constant : Constant  Value=2  OutDataTypeStr=single
  Constant1 : Constant  Value=ONEDIV3_ULS_F32  OutDataTypeStr=single
  Constant2 : Constant  Value=ONEDIVSQRT3_ULS_F32
  Constant4 : Constant  Value=ONEDIVSQRT3_ULS_F32
  CopyRight2 : Subsystem  Description=|  mask(Copyright Information){none=on}
      | Copyright info block.                                               
      |                                                                     
      | Place copyright information at the top of every subsystem in design.
      mask prompts: none "No parameters"
      mask help: Place copyright information at the top of every subsystem in design.
      mask Display:
      | NxtrConf = 'Nexteer Confidential';
      | 
      | sys = bdroot; %handle for the current model ("system")
      | first = get_param(sys,'Created');
      | first = first(end-3:end);  %year is last four digits
      | 
      | last = get_param(sys,'LastModifiedDate');
      | if isempty(last)
      |     last = datestr(now,'yyyy');
      | else
      |     last = last(end-3:end);
      | end
      | 
      | if strcmp(first,last)
      |     fprintf('%s -- Copyright %s Nexteer',NxtrConf,first)
      | else
      |     fprintf('%s -- %s%s- %s Nexteer',NxtrConf,char(169),first,last)
      | end
  Divide1 : Product  Inputs=**
  Divide2 : Product  Inputs=***
  Divide3 : Product  Inputs=****
  Divide4 : Product  Inputs=***
  Divide5 : Product  Inputs=****
  Id : Outport
  Iq : Outport  Port=2
  wires:
  Constant/1 -> Divide1/1
  A/1 -> Divide1/2
  Divide1/1 -> Add/1
  B/1 -> Add3/2, Add1/1, Add/2  "B"
  C/1 -> Add3/1, Add1/2, Add/3  "C"
  Add/1 -> Divide4/1, Divide2/1  "2A-B-C"
  Divide2/1 -> Add2/1
  Add1/1 -> Divide3/1  "B-C"
  Constant2/1 -> Divide3/2
  Divide3/1 -> Add2/2
  Add2/1 -> Id/1
  Constant1/1 -> Divide4/2, Divide2/2
  SINE/1 -> Divide3/3, Divide4/3
  Constant4/1 -> Divide5/2
  Add3/1 -> Divide5/1  "C-B"
  Add4/1 -> Iq/1
  Divide4/1 -> Add4/1
  Divide5/1 -> Add4/2
  MotCtrlMotElecMeclPolarity/1 -> Divide3/4, Divide5/4
  COS/1 -> Divide2/3, Divide5/3

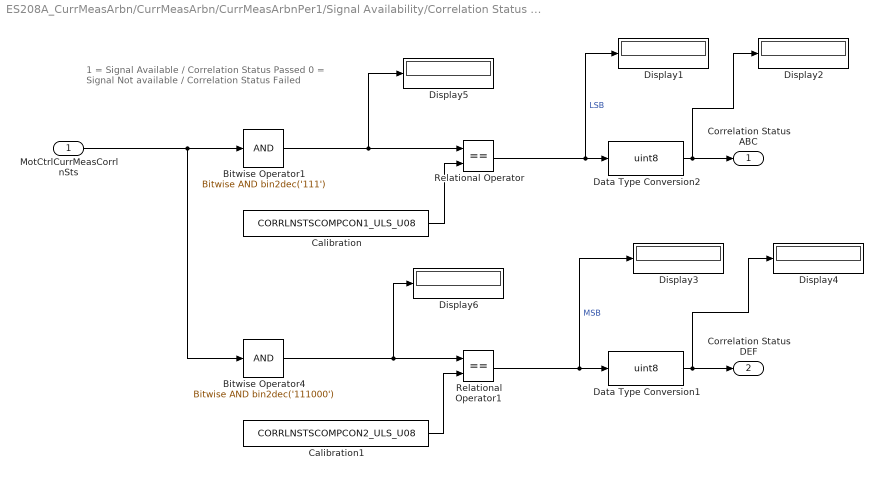
== system ES208A_CurrMeasArbn/CurrMeasArbn/CurrMeasArbnPer1/Signal Availability/Correlation Status Decomposition  ==
  note: 1 = Signal Available / Correlation Status Passed
      | 0 = Signal Not available / Correlation Status Failed
  MotCtrlCurrMeasCorrlnSts : Inport
  Bitwise Operator1 : simulink/Logic and Bit Operations/Bitwise Operator  logicop=AND  UseBitMask=on  BitMask=bin2dec('111')  BitMaskRealWorld=Stored Integer
  Bitwise Operator4 : simulink/Logic and Bit Operations/Bitwise Operator  logicop=AND  UseBitMask=on  BitMask=bin2dec('111000')  BitMaskRealWorld=Stored Integer
  Calibration : Constant  Value=CORRLNSTSCOMPCON1_ULS_U08
  Calibration1 : Constant  Value=CORRLNSTSCOMPCON2_ULS_U08
  Data Type Conversion1 : DataTypeConversion  OutDataTypeStr=uint8
  Data Type Conversion2 : DataTypeConversion  OutDataTypeStr=uint8
  Display{1..6} (6 alike) : Display
  Relational Operator : RelationalOperator  Operator===
  Relational Operator1 : RelationalOperator  Operator===
  Correlation Status ABC : Outport
  Correlation Status DEF : Outport  Port=2
  wires:
  Bitwise Operator4/1 -> Display6/1, Relational Operator1/1
  Relational Operator/1 -> Display1/1, Data Type Conversion2/1  "LSB"
  MotCtrlCurrMeasCorrlnSts/1 -> Bitwise Operator4/1, Bitwise Operator1/1
  Relational Operator1/1 -> Display3/1, Data Type Conversion1/1  "MSB"
  Bitwise Operator1/1 -> Display5/1, Relational Operator/1
  Data Type Conversion2/1 -> Correlation Status ABC/1, Display2/1
  Calibration/1 -> Relational Operator/2
  Calibration1/1 -> Relational Operator1/2
  Data Type Conversion1/1 -> Correlation Status DEF/1, Display4/1

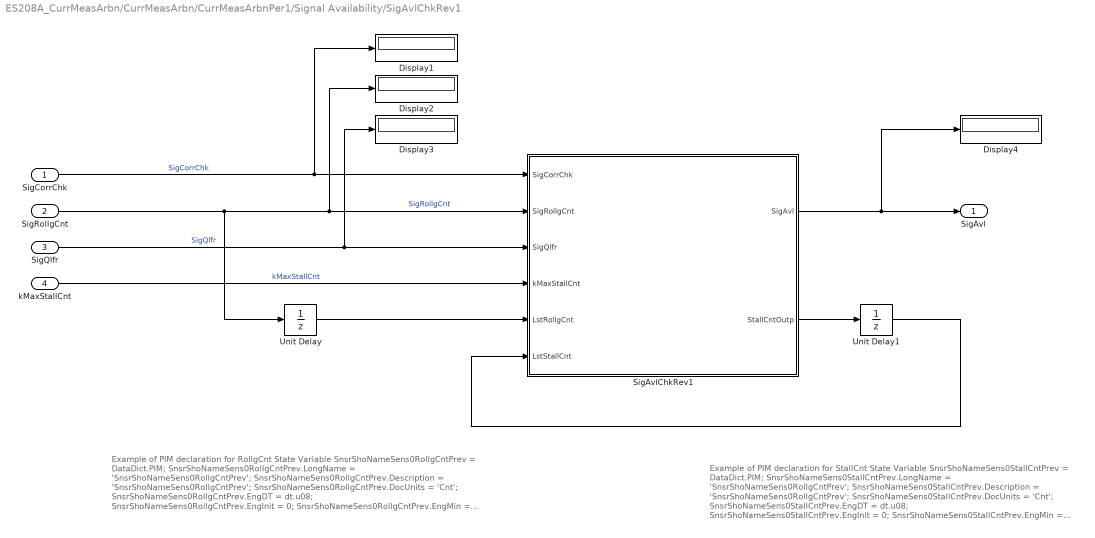
== system ES208A_CurrMeasArbn/CurrMeasArbn/CurrMeasArbnPer1/Signal Availability/SigAvlChkRev1 ==
  note: Example of PIM declaration for StallCnt State Variable
      |
      | SnsrShoNameSens0StallCntPrev = DataDict.PIM;
      | SnsrShoNameSens0StallCntPrev.LongName = 'SnsrShoNameSens0RollgCntPrev';
      | SnsrShoNameSens0StallCntPrev.Description = 'SnsrShoNameSens0RollgCntPrev';
      | SnsrShoNameSens0StallCntPrev.DocUnits = 'Cnt';
      | SnsrShoNameSens0StallCntPrev.EngDT = dt.u08;
      | SnsrShoNameSens0StallCntPrev.EngInit = 0;
      | SnsrShoNameSens0StallCntPrev.EngMin = 0;
      | SnsrShoNameSens0StallCntPrev.EngMax = 255;
      |
      |
      | *********  Need different state variable for each instance of this  subsystem ********
  note: Example of PIM declaration for RollgCnt State Variable
      |
      | SnsrShoNameSens0RollgCntPrev = DataDict.PIM;
      | SnsrShoNameSens0RollgCntPrev.LongName = 'SnsrShoNameSens0RollgCntPrev';
      | SnsrShoNameSens0RollgCntPrev.Description = 'SnsrShoNameSens0RollgCntPrev';
      | SnsrShoNameSens0RollgCntPrev.DocUnits = 'Cnt';
      | SnsrShoNameSens0RollgCntPrev.EngDT = dt.u08;
      | SnsrShoNameSens0RollgCntPrev.EngInit = 0;
      | SnsrShoNameSens0RollgCntPrev.EngMin = 0;
      | SnsrShoNameSens0RollgCntPrev.EngMax = 255;
      |
      |
      | *********  Need different state variable for each instance of this  subsystem ********
  SigCorrChk : Inport  OutDataTypeStr=uint8
  SigRollgCnt : Inport  Port=2  OutDataTypeStr=uint8
  SigQlfr : Inport  Port=3  OutDataTypeStr=uint8
  kMaxStallCnt : Inport  Port=4  OutDataTypeStr=uint8
  Display{1..4} (4 alike) : Display
  SigAvlChkRev1 : Stateflow chart  TreatAsAtomicUnit=on
  Unit Delay : UnitDelay  SampleTime=-1  StateName=ArbnSnsr0RollgCntPrev  StateMustResolveToSignalObject=on
      settings: AttributesFormatString=|
      | State Variable:
      | %<StateName>
  Unit Delay1 : UnitDelay  SampleTime=-1  StateName=ArbnSnsr0StallCntPrev  StateMustResolveToSignalObject=on
      settings: AttributesFormatString=|
      | State Variable:
      | %<StateName>
  SigAvl : Outport
  wires:
  SigCorrChk/1 -> Display1/1, SigAvlChkRev1/1(SigCorrChk)  "SigCorrChk"
  SigRollgCnt/1 -> Unit Delay/1, Display2/1, SigAvlChkRev1/2(SigRollgCnt)  "SigRollgCnt"
  SigQlfr/1 -> Display3/1, SigAvlChkRev1/3(SigQlfr)  "SigQlfr"
  kMaxStallCnt/1 -> SigAvlChkRev1/4(kMaxStallCnt)  "kMaxStallCnt"
  Unit Delay/1 -> SigAvlChkRev1/5(LstRollgCnt)
  SigAvlChkRev1/2(StallCntOutp) -> Unit Delay1/1
  Unit Delay1/1 -> SigAvlChkRev1/6(LstStallCnt)
  SigAvlChkRev1/1(SigAvl) -> Display4/1, SigAvl/1

== system ES208A_CurrMeasArbn/CurrMeasArbn/CurrMeasArbnPer1/Signal Availability/SigAvlChkRev2 ==
  note: Example of PIM declaration for StallCnt State Variable
      |
      | SnsrShoNameSens0StallCntPrev = DataDict.PIM;
      | SnsrShoNameSens0StallCntPrev.LongName = 'SnsrShoNameSens0RollgCntPrev';
      | SnsrShoNameSens0StallCntPrev.Description = 'SnsrShoNameSens0RollgCntPrev';
      | SnsrShoNameSens0StallCntPrev.DocUnits = 'Cnt';
      | SnsrShoNameSens0StallCntPrev.EngDT = dt.u08;
      | SnsrShoNameSens0StallCntPrev.EngInit = 0;
      | SnsrShoNameSens0StallCntPrev.EngMin = 0;
      | SnsrShoNameSens0StallCntPrev.EngMax = 255;
      |
      |
      | *********  Need different state variable for each instance of this  subsystem ********
  note: Example of PIM declaration for RollgCnt State Variable
      |
      | SnsrShoNameSens0RollgCntPrev = DataDict.PIM;
      | SnsrShoNameSens0RollgCntPrev.LongName = 'SnsrShoNameSens0RollgCntPrev';
      | SnsrShoNameSens0RollgCntPrev.Description = 'SnsrShoNameSens0RollgCntPrev';
      | SnsrShoNameSens0RollgCntPrev.DocUnits = 'Cnt';
      | SnsrShoNameSens0RollgCntPrev.EngDT = dt.u08;
      | SnsrShoNameSens0RollgCntPrev.EngInit = 0;
      | SnsrShoNameSens0RollgCntPrev.EngMin = 0;
      | SnsrShoNameSens0RollgCntPrev.EngMax = 255;
      |
      |
      | *********  Need different state variable for each instance of this  subsystem ********
  SigCorrChk : Inport  OutDataTypeStr=uint8
  SigRollgCnt : Inport  Port=2  OutDataTypeStr=uint8
  SigQlfr : Inport  Port=3  OutDataTypeStr=uint8
  kMaxStallCnt : Inport  Port=4  OutDataTypeStr=uint8
  SigAvlChkRev1 : Stateflow chart  TreatAsAtomicUnit=on
  Unit Delay : UnitDelay  SampleTime=-1  StateName=ArbnSnsr1RollgCntPrev  StateMustResolveToSignalObject=on
      settings: AttributesFormatString=|
      | State Variable:
      | %<StateName>
  Unit Delay1 : UnitDelay  SampleTime=-1  StateName=ArbnSnsr1StallCntPrev  StateMustResolveToSignalObject=on
      settings: AttributesFormatString=|
      | State Variable:
      | %<StateName>
  SigAvl : Outport
  wires:
  SigCorrChk/1 -> SigAvlChkRev1/1(SigCorrChk)  "SigCorrChk"
  SigRollgCnt/1 -> Unit Delay/1, SigAvlChkRev1/2(SigRollgCnt)  "SigRollgCnt"
  SigQlfr/1 -> SigAvlChkRev1/3(SigQlfr)  "SigQlfr"
  kMaxStallCnt/1 -> SigAvlChkRev1/4(kMaxStallCnt)  "kMaxStallCnt"
  Unit Delay/1 -> SigAvlChkRev1/5(LstRollgCnt)
  SigAvlChkRev1/2(StallCntOutp) -> Unit Delay1/1
  Unit Delay1/1 -> SigAvlChkRev1/6(LstStallCnt)
  SigAvlChkRev1/1(SigAvl) -> SigAvl/1

== system ES208A_CurrMeasArbn/CurrMeasArbn/CurrMeasArbnPer1/Switch Case Action Subsyste - Case 0/CopyRight2 ==

== system ES208A_CurrMeasArbn/CurrMeasArbn/CurrMeasArbnPer1/Switch Case Action Subsyste - Case 3/CopyRight2 ==

== system ES208A_CurrMeasArbn/CurrMeasArbn/CurrMeasArbnPer1/Switch Case Action Subsystem - Case 1/Average ==
  In1 : Inport
  In2 : Inport  Port=2
  Add : Sum
  Constant : Constant  Value=2  OutDataTypeStr=single
  Divide : Product  Inputs=*/
  Out1 : Outport
  wires:
  In1/1 -> Add/1
  In2/1 -> Add/2
  Add/1 -> Divide/1
  Constant/1 -> Divide/2
  Divide/1 -> Out1/1

== system ES208A_CurrMeasArbn/CurrMeasArbn/CurrMeasArbnPer1/Switch Case Action Subsystem - Case 1/Average1 ==
  In1 : Inport
  In2 : Inport  Port=2
  Add : Sum
  Constant : Constant  Value=2  OutDataTypeStr=single
  Divide : Product  Inputs=*/
  Out1 : Outport
  wires:
  Divide/1 -> Out1/1
  Constant/1 -> Divide/2
  Add/1 -> Divide/1
  In2/1 -> Add/2
  In1/1 -> Add/1

== system ES208A_CurrMeasArbn/CurrMeasArbn/CurrMeasArbnPer1/Switch Case Action Subsystem - Case 1/Average2 ==
  In1 : Inport
  In2 : Inport  Port=2
  Add : Sum
  Constant : Constant  Value=2  OutDataTypeStr=single
  Divide : Product  Inputs=*/
  Out1 : Outport
  wires:
  In1/1 -> Add/1
  In2/1 -> Add/2
  Add/1 -> Divide/1
  Constant/1 -> Divide/2
  Divide/1 -> Out1/1

== system ES208A_CurrMeasArbn/CurrMeasArbn/CurrMeasArbnPer1/Switch Case Action Subsystem - Case 1/CopyRight2 ==

== system ES208A_CurrMeasArbn/CurrMeasArbn/CurrMeasArbnPer1/Switch Case Action Subsystem - Case 2/CopyRight2 ==

== system ES208A_CurrMeasArbn/CurrMeasArbn/CurrMeasArbnPer1/Calculate Id, Iq/Park transformation/CopyRight2 ==

== stateflow chart ES208A_CurrMeasArbn/CurrMeasArbn/CurrMeasArbnPer1/Signal Availability/SigAvlChkRev1/SigAvlChkRev1 ==
  note: SigAvl
      | False = 0
      | Pass = 1
  note: SigQlfr
      | 0 = No Result
      | 1 = Pass
      | 2 = Fail
  (default) -> (junction 89)
  (junction 89) -> (junction 76) [order 1] : [SigRollgCnt ==LstRollgCnt]
  (junction 76) -> (junction 69) [order 2] : {
      | StallCntOutp = LstStallCnt +1;
      | }
  (junction 89) -> (junction 82) [order 2]
  (junction 76) -> (junction 69) [order 1] : [LstStallCnt == 255]
      | {
      | StallCntOutp = 255;
      | }
  (junction 82) -> (junction 69) : {
      | StallCntOutp = 0;
      | }
  (junction 69) -> (junction 67)
  (junction 67) -> (junction 86) [order 1] : [StallCntOutp >=kMaxStallCnt]
  (junction 67) -> (junction 78) [order 2]
  (junction 86) -> (junction 74)
  (junction 78) -> (junction 74) [order 2]
  (junction 78) -> (junction 79) [order 1] : [SigQlfr<2 && SigCorrChk>=1]
  (junction 74) -> (junction 83) : {
      | SigAvl =0;
      | }
  (junction 79) -> (junction 83) : {
      | SigAvl = 1;
      | }
  data: SigCorrChk input uint8; SigRollgCnt input; SigQlfr input; kMaxStallCnt input; SigAvl output uint8; LstRollgCnt input uint8; LstStallCnt input uint8; StallCntOutp output uint8

== matlab function ES208A_CurrMeasArbn/CurrMeasArbn/CurrMeasArbnPer1/Truth Table1 ==
  data: u2 input; y output; u1 input
function y = fcn(u2, u1)

aVarTruthTableCondition_1 = false;
aVarTruthTableCondition_2 = false;


% ABC = 1

aVarTruthTableCondition_1 = logical(u2 == 1);

% DEF = 1

aVarTruthTableCondition_2 = logical(u1 == 1);

if (~aVarTruthTableCondition_1 && ~aVarTruthTableCondition_2)
    aFcnTruthTableAction_4();
elseif (~aVarTruthTableCondition_1 && aVarTruthTableCondition_2)
    aFcnTruthTableAction_2();
elseif (aVarTruthTableCondition_1 && ~aVarTruthTableCondition_2)
    aFcnTruthTableAction_3();
else % Default
    aFcnTruthTableAction_1();
end

function aFcnTruthTableAction_1()

% Action 1

y = 1;

function aFcnTruthTableAction_2()

% Action 2

y = 2;

function aFcnTruthTableAction_3()

% Action 3

y = 3;

function aFcnTruthTableAction_4()

% Default

y = 0;

== stateflow chart ES208A_CurrMeasArbn/CurrMeasArbn/CurrMeasArbnPer1/Signal Availability/SigAvlChkRev2/SigAvlChkRev1 ==
  note: SigAvl
      | False = 0
      | Pass = 1
  note: SigQlfr
      | 0 = No Result
      | 1 = Pass
      | 2 = Fail
  (default) -> (junction 99)
  (junction 99) -> (junction 86) [order 1] : [SigRollgCnt ==LstRollgCnt]
  (junction 86) -> (junction 79) [order 2] : {
      | StallCntOutp = LstStallCnt +1;
      | }
  (junction 99) -> (junction 92) [order 2]
  (junction 86) -> (junction 79) [order 1] : [LstStallCnt == 255]
      | {
      | StallCntOutp = 255;
      | }
  (junction 92) -> (junction 79) : {
      | StallCntOutp = 0;
      | }
  (junction 79) -> (junction 77)
  (junction 77) -> (junction 96) [order 1] : [StallCntOutp >=kMaxStallCnt]
  (junction 77) -> (junction 88) [order 2]
  (junction 96) -> (junction 84)
  (junction 88) -> (junction 84) [order 2]
  (junction 88) -> (junction 89) [order 1] : [SigQlfr<2 && SigCorrChk>=1]
  (junction 84) -> (junction 93) : {
      | SigAvl =0;
      | }
  (junction 89) -> (junction 93) : {
      | SigAvl = 1;
      | }
  data: SigCorrChk input uint8; SigRollgCnt input; SigQlfr input; kMaxStallCnt input; SigAvl output uint8; LstRollgCnt input uint8; LstStallCnt input uint8; StallCntOutp output uint8
